simulink model "MASH"  (R2025b)
settings: Solver=VariableStepAuto  StartTime=0.0  StopTime=4.608  RelTol=1e-9
undefined symbols (not defined in the file): designMultirateFIR
libraries: msbAdcFoundation x2, dspquant2 x2, msbAdcMeasurements x1, dspmlti4 x1, dspfdesign x1
settings Model: Creator=The MathWorks, Inc.  LastModifiedBy=sohom
settings RTWCC: LargeConstantGeneration=WriteOnlyDNNConstantsToDataFiles

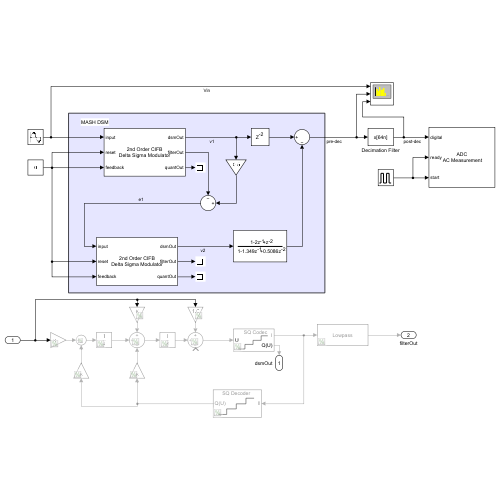
[thumbnail: Simulink's stored preview of the top-level diagram]
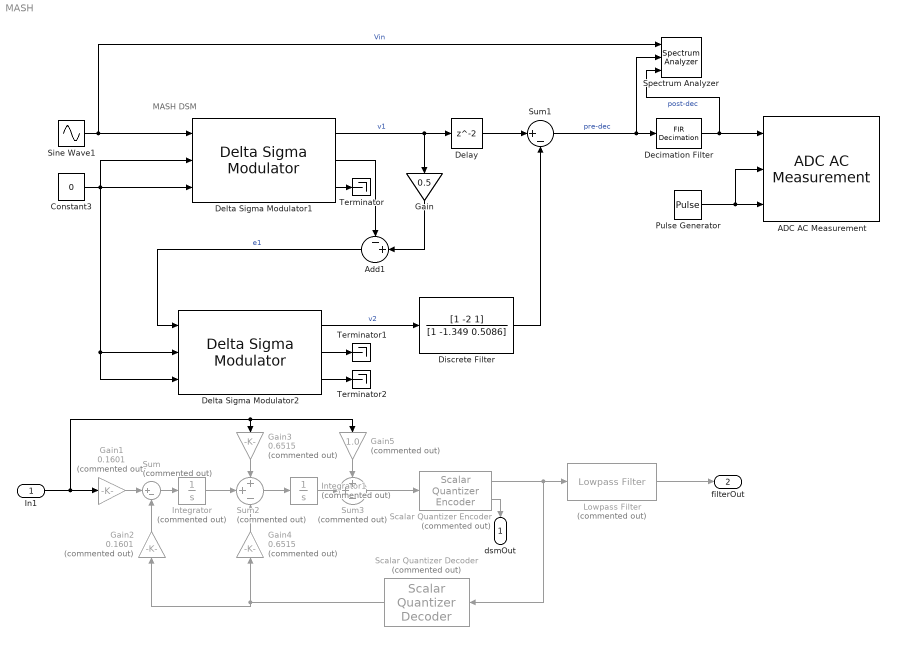
== system MASH ==
  note: MASH DSM
  In1 : Inport
  ADC AC Measurement : msbAdcMeasurements/ADC AC Measurement  DistortionMeasurement=Harmonic  InputFrequency=900  Method=Welch (faster, potentially more leakage)  RBW=1.9531  AutoSetRBW=on  NBits=5  Frequency=2e3  HoldOffTime=0  OutputToWorkspace=on  VariableName=mash_ac_out  ShowSpectrum=off
  Add1 : Sum  Inputs=-+|
  Constant3 : Constant  Value=0
  Decimation Filter : dspmlti4/FIR Decimation  FilterSource=Auto  h=designMultirateFIR(1,2)  D=64  filtStruct=Direct form  FilterObject=FDECIM  framing=Allow multirate processing  AllowArbitraryInputLength=off  inputOffset=0  outputBufInitCond=0  roundingMode=Floor  overflowMode=off  firstCoeffDataTypeStr=Inherit: Same word length as input  firstCoeffMin=[]  firstCoeffMax=[]  firstCoeffLastDataTypeStr=Inherit: Same word length as input  outputDataTypeStr=Inherit: Same as accumulator  outputMin=[]  outputMax=[]  outputLastDataTypeStr=Inherit: Same as accumulator
      settings: LibrarySourceBlock=|
      | dsphdlsupportfiltering/FIR
      | Decimation
  Delay : Delay
  Delta Sigma Modulator1 : msbAdcFoundation/Delta Sigma Modulator  dsmArchitecture=CIFB  dsmOrder=2nd order  BandWidth=1000  OSR=64  SamplingFrequency=128000  NumberLevels=2  QuantizerOutput=-1:2:1  BoundaryPoints=[-1:1:1]  EnableDynamicRangeScaling=off  EnableCustomCoeff=off  a=[0.1601 0.6515]  g=[0.0000]  b=[0.1601 0.6515 1.0000]  c=[1.0000 1.0000]  OLgain=Inf  EnableNoise=off  thermalNoiseValue=200e-6  thermalNoiseUnit=Vrms  refResistance=50  wNoiseGain=0.0002  fcorner=1000  pNoiseGain=5e-06  ntfOptim=2: Optimized with at least one zero at band-center  passbandType=Lowpass  centerFrequency=0  EnableCustomHinf=off  Hinf=1.4  NTFflag=on  PZflag=off  STFflag=off  SNRflag=off  AppendFlag=off  ExportFlag=off
      link override Delta Sigma Modulator: LabelModeActiveChoice=2CIFB
      link override Noise: LabelModeActiveChoice=noNoise
  Delta Sigma Modulator2 : msbAdcFoundation/Delta Sigma Modulator  dsmArchitecture=CIFB  dsmOrder=2nd order  BandWidth=1000  OSR=64  SamplingFrequency=128000  NumberLevels=2  QuantizerOutput=-1:2:1  BoundaryPoints=[-1:1:1]  EnableDynamicRangeScaling=off  EnableCustomCoeff=off  a=[0.1601 0.6515]  g=[0.0000]  b=[0.1601 0.6515 1.0000]  c=[1.0000 1.0000]  OLgain=Inf  EnableNoise=off  thermalNoiseValue=200e-6  thermalNoiseUnit=Vrms  refResistance=50  wNoiseGain=0.0002  fcorner=1000  pNoiseGain=5e-06  ntfOptim=2: Optimized with at least one zero at band-center  passbandType=Lowpass  centerFrequency=0  EnableCustomHinf=off  Hinf=1.4  NTFflag=on  PZflag=off  STFflag=off  SNRflag=off  AppendFlag=off  ExportFlag=off
      link override Delta Sigma Modulator: LabelModeActiveChoice=2CIFB
      link override Noise: LabelModeActiveChoice=noNoise
  Discrete Filter : DiscreteFilter  Numerator=[1 -2 1]  Denominator=[1 -1.349 0.5086]
  Gain : Gain  Gain=0.5
  Gain1 : Gain  Commented=on  Gain=0.1601
  Gain2 : Gain  Commented=on  Gain=0.1601
  Gain3 : Gain  Commented=on  Gain=0.6515
  Gain4 : Gain  Commented=on  Gain=0.6515
  Gain5 : Gain  Commented=on  Gain=1.0
  Integrator : Integrator  Commented=on
  Integrator1 : Integrator  Commented=on
  Lowpass Filter : dspfdesign/Lowpass Filter  Commented=on  FilterType=FIR  DesignForMinimumOrder=on  FilterOrder=50  PassbandFrequency=1000  StopbandFrequency=3000  PassbandRipple=0.1  StopbandAttenuation=80  SampleRateMode=Specify on dialog  SampleRate=128000  SimulateUsing=Interpreted execution  roundingMode=Floor  coeffsDataTypeStr=fixdt(1,16)
  Pulse Generator : DiscretePulseGenerator  PulseType=Time based  Period=1/2e3  PulseWidth=50
  Scalar Quantizer Decoder : dspquant2/Scalar Quantizer Decoder  Commented=on  invalidin=Clip  CBsource=Specify via dialog  codebook=[1:10]  dataType=double  isSigned=on  wordLen=16  udDataType=sfix(16)  fracBitsMode=Best precision  numFracBits=11  OutDataTypeStr=double  LastOutDataTypeStr=double
  Scalar Quantizer Encoder : dspquant2/Scalar Quantizer Encoder  Commented=on  paramSrc=Specify via dialog  partType=Bounded  BBoundary=[1:10]  UBoundary=[2:9]  SearchMethod=Linear  tieBreakRule=Choose the lower index  outQU=on  outQError=off  codebook=[1.5:9.5]  outStatus=off  invalidin=Clip  idtype=int32  roundingMode=Floor  overflowMode=off
  Sine Wave1 : Sin  Amplitude=0.7  Frequency=2*pi*0.9e3  Phase=pi  SampleTime=1/128e3
  Spectrum Analyzer : SpectrumAnalyzer  NumInputPorts=3  WindowPosition=[42.000000,33.000000,1209.000000,591.000000,]  Visible=on  ScopeFrameLocation=window  SpectrumType=Power density  SampleRate=44.1e3  PlotAsTwoSidedSpectrum=off  FrequencyScale=Log  StartFrequency=20  StopFrequency=20e3  SpectrumUnits=dBm/Hz  YLimits=[-218.6793 29.1967]  ShowLegend=on
  Sum : Sum  Commented=on  Inputs=|+-
  Sum1 : Sum  Inputs=|+-
  Sum2 : Sum  Commented=on  Inputs=++-
  Sum3 : Sum  Commented=on  Inputs=++-
  Terminator : Terminator
  Terminator1 : Terminator
  Terminator2 : Terminator
  dsmOut : Outport
  filterOut : Outport  Port=2
  wires:
  Delta Sigma Modulator1/1 -> Gain/1, Delay/1  "v1"
  Delay/1 -> Sum1/1
  Constant3/1 -> Delta Sigma Modulator1/2, Delta Sigma Modulator2/2, Delta Sigma Modulator2/3, Delta Sigma Modulator1/3
  Delta Sigma Modulator2/2 -> Terminator1/1
  Sum1/1 -> Spectrum Analyzer/2, Decimation Filter/1  "pre-dec"
  Delta Sigma Modulator1/2 -> Add1/1
  Delta Sigma Modulator1/3 -> Terminator/1
  Delta Sigma Modulator2/3 -> Terminator2/1
  Gain/1 -> Add1/2
  Sine Wave1/1 -> Spectrum Analyzer/1, Delta Sigma Modulator1/1  "Vin"
  Pulse Generator/1 -> ADC AC Measurement/3, ADC AC Measurement/2
  Decimation Filter/1 -> Spectrum Analyzer/3, ADC AC Measurement/1  "post-dec"
  Delta Sigma Modulator2/1 -> Discrete Filter/1  "v2"
  Discrete Filter/1 -> Sum1/2
  Add1/1 -> Delta Sigma Modulator2/1  "e1"
  Sum/1 -> Integrator/1
  Gain1/1 -> Sum/1
  Gain2/1 -> Sum/2
  Sum2/1 -> Integrator1/1
  Integrator/1 -> Sum2/2
  Gain3/1 -> Sum2/1
  In1/1 -> Gain5/1, Gain3/1, Gain1/1
  Gain4/1 -> Sum2/3
  Scalar Quantizer Encoder/1 -> Scalar Quantizer Decoder/1, Lowpass Filter/1
  Scalar Quantizer Decoder/1 -> Gain2/1, Gain4/1
  Scalar Quantizer Encoder/2 -> dsmOut/1
  Lowpass Filter/1 -> filterOut/1
  Integrator1/1 -> Sum3/2
  Sum3/1 -> Scalar Quantizer Encoder/1
  Gain5/1 -> Sum3/1
